simulink model "model_1"  (R2021b)
settings: Solver=VariableStepAuto  StartTime=0.0  StopTime=10  RelTol=1e-3
values from neighbouring files (symbols this model uses):
  A = [-6, -25, -35, -10; 0, -9, -15, 0; 0, 6, 9, 0; 4, 17, 26, 6]    [task_1.m]    (also in task_2.m; task_3.m; task_4.m)
  B = [16, 0; 3, 0; -3, 0; -11, 0]    [task_1.m]    (also in task_2.m; task_3.m = [0; 0; 0; 0]; task_4.m)
  C = eye(4)    [task_1.m]    (also in task_2.m; task_3.m = [2, 2, 0, 4; 0, 3, 6, 0]; task_4.m = [2, 2, 0, 4; 0, 3, 6, 0])
  D = zeros(4, 2)    [task_1.m]    (also in task_2.m; task_3.m = zeros(2, 1); task_4.m = [0, 0; 0, 4])
  K_1 = -K_1    [task_1.m]    (also in task_2.m)
  K_2 = -K_2    [task_1.m]    (also in task_2.m = Y*inv(P))
  K_3 = -K_3    [task_1.m]    (also in task_2.m = Y*inv(P))
  x0 = [1000; -1000; 1000; -1000]    [task_1.m]    (also in task_2.m; task_3.m = [10; -10; 5; -5]; task_4.m = [10; -10; 5; -5])
settings Model: Creator=vital  LastModifiedBy=vital

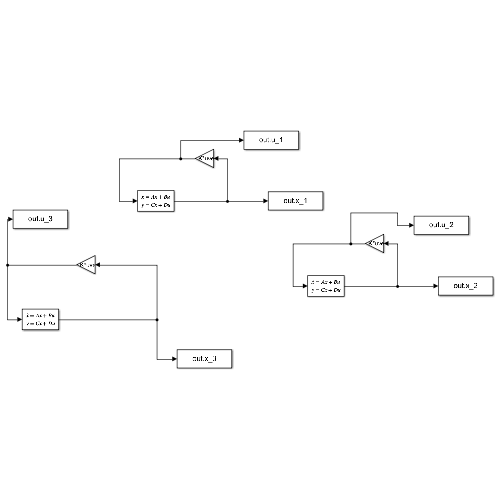
[thumbnail: Simulink's stored preview of the top-level diagram]
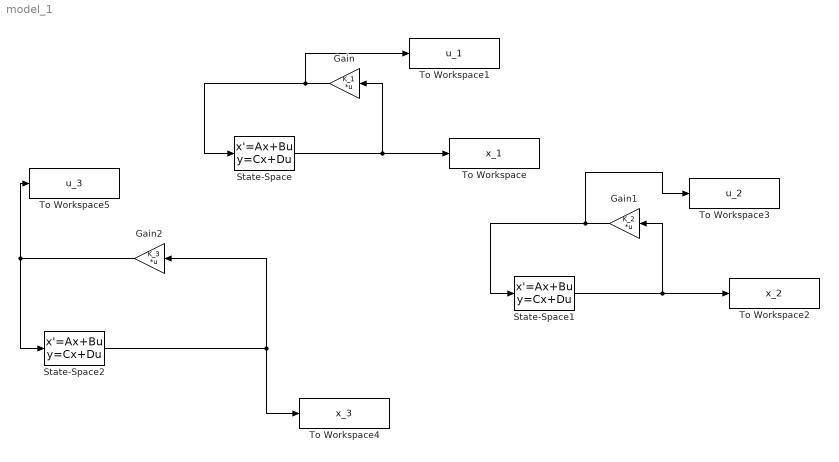
== system model_1 ==
  Gain : Gain  Gain=K_1  Multiplication=Matrix(K*u) (u vector)
  Gain1 : Gain  Gain=K_2  Multiplication=Matrix(K*u) (u vector)
  Gain2 : Gain  Gain=K_3  Multiplication=Matrix(K*u) (u vector)
  State-Space : StateSpace  A=A  B=B  C=C  D=D  InitialCondition=x0  ParameterTunability=Optimized
  State-Space1 : StateSpace  A=A  B=B  C=C  D=D  InitialCondition=x0  ParameterTunability=Unconstrained
  State-Space2 : StateSpace  A=A  B=B  C=C  D=D  InitialCondition=x0  ParameterTunability=Optimized
  To Workspace : ToWorkspace  VariableName=x_1  SaveFormat=Timeseries  SampleTime=-1
  To Workspace1 : ToWorkspace  VariableName=u_1  SaveFormat=Timeseries  SampleTime=0.00001
  To Workspace2 : ToWorkspace  VariableName=x_2  SaveFormat=Timeseries  SampleTime=-1
  To Workspace3 : ToWorkspace  VariableName=u_2  SaveFormat=Timeseries  SampleTime=0.00001
  To Workspace4 : ToWorkspace  VariableName=x_3  SaveFormat=Timeseries  SampleTime=-1
  To Workspace5 : ToWorkspace  VariableName=u_3  SaveFormat=Timeseries  SampleTime=0.00001
  wires:
  State-Space/1 -> Gain/1, To Workspace/1
  State-Space2/1 -> Gain2/1, To Workspace4/1
  Gain1/1 -> To Workspace3/1, State-Space1/1
  State-Space1/1 -> Gain1/1, To Workspace2/1
  Gain/1 -> To Workspace1/1, State-Space/1
  Gain2/1 -> To Workspace5/1, State-Space2/1
